simulink model "examples_of_gain"  (R2021a)
settings: Solver=VariableStepAuto  StartTime=0.0  StopTime=1  RelTol=1e-3
settings Model: Creator=YasserNet  LastModifiedBy=YasserNet

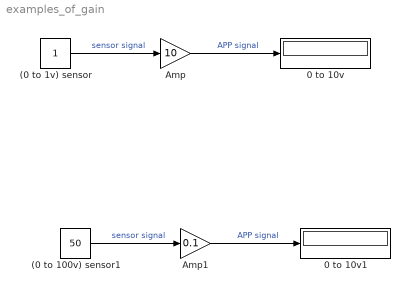
== system examples_of_gain ==
  (0 to 100v) sensor1 : Constant  Value=50
  (0 to 1v) sensor : Constant
  0 to 10v : Display
  0 to 10v1 : Display
  Amp : Gain  Gain=10
  Amp1 : Gain  Gain=0.1
  wires:
  (0 to 1v) sensor/1 -> Amp/1  "sensor signal"
  Amp/1 -> 0 to 10v/1  "APP signal"
  (0 to 100v) sensor1/1 -> Amp1/1  "sensor signal"
  Amp1/1 -> 0 to 10v1/1  "APP signal"
